simulink model "Project_microgrid_2018a"  (Simulink 9.1)
settings: Solver=VariableStepAuto  StartTime=0.0  StopTime=0.3  RelTol=1e-3
undefined symbols (not defined in the file): D1, D11, Delta, DiscIntNeverNeededParam, find_system, Hydride, Metal, Nickel
libraries: powerlib x104, powerlib_meascontrol x31, sps_avr x14, simulink_extras x4, simulink x3, spsDieselMotorModel x2, electricdrivelib x1, re_lib x1
(part 2 of 5)

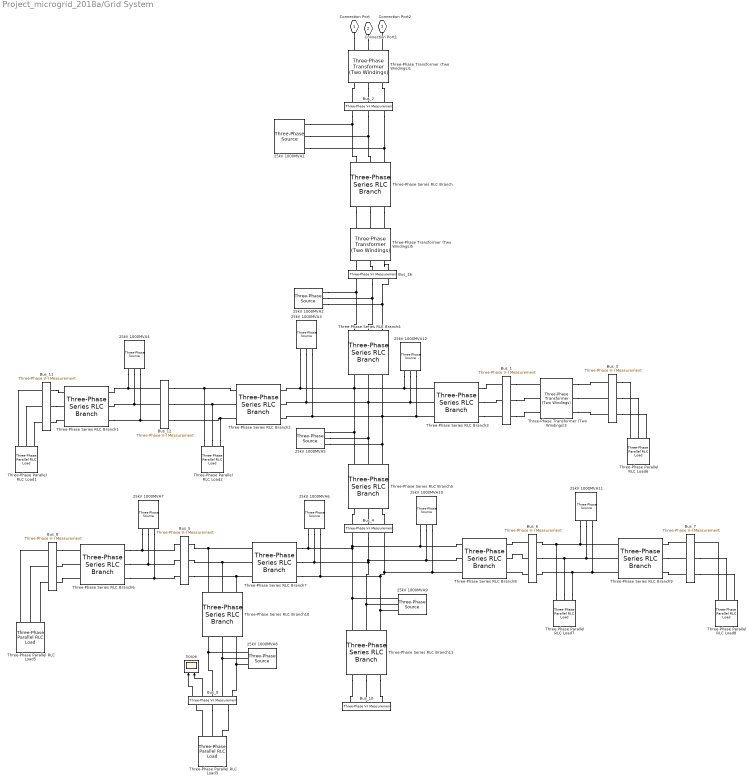
== system Project_microgrid_2018a/Grid System ==
  25kV 1000MVA{1..4,6..12} (11 alike) : powerlib/Electrical Sources/Three-Phase Source  InternalConnection=Yg  VoltagePhases=off  Voltage=10  PhaseAngle=0  Voltage_phases=[25e3 25e3 25e3]/sqrt(3)  PhaseAngles_phases=[0 -120 +120]  Frequency=50  NonIdealSource=on  SpecifyImpedance=on  Resistance=25^2/1000/10  Inductance=25^2/1000/377  ShortCircuitLevel=1000e6  BaseVoltage=25e3  XRratio=10  BusType=swing  Pref=10e3  Qref=0  Prefabc=[10e3, 10e3, 10e3]  Qrefabc=[0, 0, 0]  Qmin=-inf  Qmax=inf
      settings: SourceProductName=Simscape Electrical
  25kV 1000MVA5 : powerlib/Electrical Sources/Three-Phase Source  InternalConnection=Yg  VoltagePhases=off  Voltage=25e3  PhaseAngle=0  Voltage_phases=[25e3 25e3 25e3]/sqrt(3)  PhaseAngles_phases=[0 -120 +120]  Frequency=50  NonIdealSource=on  SpecifyImpedance=on  Resistance=25^2/1000/10  Inductance=25^2/1000/377  ShortCircuitLevel=1000e6  BaseVoltage=25e3  XRratio=10  BusType=swing  Pref=10e3  Qref=0  Prefabc=[10e3, 10e3, 10e3]  Qrefabc=[0, 0, 0]  Qmin=-inf  Qmax=inf
      settings: SourceProductName=Simscape Electrical
  Bus_1 : powerlib/Measurements/Three-Phase V-I Measurement  VoltageMeasurement=phase-to-phase  SetLabelV=on  LabelV=Vabc_5  Vpu=off  VpuLL=off  CurrentMeasurement=yes  SetLabelI=on  LabelI=Iabc_5  Ipu=off  Pbase=100e6  Vbase=120e3  OutputType=Complex  PhasorSimulation=on  PSBequivalent=0
      settings: SourceProductName=Simscape Electrical
  Bus_10 : powerlib/Measurements/Three-Phase V-I Measurement  VoltageMeasurement=phase-to-phase  SetLabelV=on  LabelV=Vabc_13  Vpu=off  VpuLL=off  CurrentMeasurement=yes  SetLabelI=on  LabelI=Iabc_13  Ipu=off  Pbase=100e6  Vbase=120e3  OutputType=Complex  PhasorSimulation=on  PSBequivalent=0
      settings: SourceProductName=Simscape Electrical
  Bus_11 : powerlib/Measurements/Three-Phase V-I Measurement  VoltageMeasurement=phase-to-phase  SetLabelV=on  LabelV=Vabc_3  Vpu=off  VpuLL=off  CurrentMeasurement=yes  SetLabelI=on  LabelI=Iabc_3  Ipu=off  Pbase=100e6  Vbase=120e3  OutputType=Complex  PhasorSimulation=on  PSBequivalent=0
      settings: SourceProductName=Simscape Electrical
  Bus_12 : powerlib/Measurements/Three-Phase V-I Measurement  VoltageMeasurement=phase-to-phase  SetLabelV=on  LabelV=Vabc_4  Vpu=off  VpuLL=off  CurrentMeasurement=yes  SetLabelI=on  LabelI=Iabc_4  Ipu=off  Pbase=100e6  Vbase=120e3  OutputType=Complex  PhasorSimulation=on  PSBequivalent=0
      settings: SourceProductName=Simscape Electrical
  Bus_16 : powerlib/Measurements/Three-Phase V-I Measurement  VoltageMeasurement=phase-to-phase  SetLabelV=on  LabelV=Vabc_1  Vpu=off  VpuLL=off  CurrentMeasurement=yes  SetLabelI=on  LabelI=Iabc_1  Ipu=off  Pbase=100e6  Vbase=120e3  OutputType=Complex  PhasorSimulation=on  PSBequivalent=0
      settings: SourceProductName=Simscape Electrical
  Bus_2 : powerlib/Measurements/Three-Phase V-I Measurement  VoltageMeasurement=phase-to-phase  SetLabelV=on  LabelV=Vabc_2  Vpu=off  VpuLL=off  CurrentMeasurement=yes  SetLabelI=on  LabelI=Iabc_2  Ipu=off  Pbase=100e6  Vbase=120e3  OutputType=Complex  PhasorSimulation=on  PSBequivalent=0
      settings: SourceProductName=Simscape Electrical
  Bus_3 : powerlib/Measurements/Three-Phase V-I Measurement  VoltageMeasurement=phase-to-phase  SetLabelV=on  LabelV=Vabc_6  Vpu=off  VpuLL=off  CurrentMeasurement=yes  SetLabelI=on  LabelI=Iabc_6  Ipu=off  Pbase=100e6  Vbase=120e3  OutputType=Complex  PhasorSimulation=on  PSBequivalent=0
      settings: SourceProductName=Simscape Electrical
  Bus_4 : powerlib/Measurements/Three-Phase V-I Measurement  VoltageMeasurement=phase-to-phase  SetLabelV=on  LabelV=Vabc_7  Vpu=off  VpuLL=off  CurrentMeasurement=yes  SetLabelI=on  LabelI=Iabc_7  Ipu=off  Pbase=100e6  Vbase=120e3  OutputType=Complex  PhasorSimulation=on  PSBequivalent=0
      settings: SourceProductName=Simscape Electrical
  Bus_5 : powerlib/Measurements/Three-Phase V-I Measurement  VoltageMeasurement=phase-to-phase  SetLabelV=on  LabelV=Vabc_8  Vpu=off  VpuLL=off  CurrentMeasurement=yes  SetLabelI=on  LabelI=Iabc_8  Ipu=off  Pbase=100e6  Vbase=120e3  OutputType=Complex  PhasorSimulation=on  PSBequivalent=0
      settings: SourceProductName=Simscape Electrical
  Bus_6 : powerlib/Measurements/Three-Phase V-I Measurement  VoltageMeasurement=phase-to-phase  SetLabelV=on  LabelV=Vabc_10  Vpu=off  VpuLL=off  CurrentMeasurement=yes  SetLabelI=on  LabelI=Iabc_10  Ipu=off  Pbase=100e6  Vbase=120e3  OutputType=Complex  PhasorSimulation=on  PSBequivalent=0
      settings: SourceProductName=Simscape Electrical
  Bus_7 : powerlib/Measurements/Three-Phase V-I Measurement  VoltageMeasurement=phase-to-phase  SetLabelV=on  LabelV=Vabc_11  Vpu=off  VpuLL=off  CurrentMeasurement=yes  SetLabelI=on  LabelI=Iabc_11  Ipu=off  Pbase=100e6  Vbase=120e3  OutputType=Complex  PhasorSimulation=on  PSBequivalent=0
      settings: SourceProductName=Simscape Electrical
  Bus_8 : powerlib/Measurements/Three-Phase V-I Measurement  VoltageMeasurement=phase-to-phase  SetLabelV=on  LabelV=Vabc_9  Vpu=off  VpuLL=off  CurrentMeasurement=yes  SetLabelI=on  LabelI=Iabc_9  Ipu=off  Pbase=100e6  Vbase=120e3  OutputType=Complex  PhasorSimulation=on  PSBequivalent=0
      settings: SourceProductName=Simscape Electrical
  Bus_9 : powerlib/Measurements/Three-Phase V-I Measurement  VoltageMeasurement=phase-to-phase  SetLabelV=off  LabelV=Vabc_12  Vpu=off  VpuLL=off  CurrentMeasurement=yes  SetLabelI=off  LabelI=Iabc_12  Ipu=off  Pbase=100e6  Vbase=120e3  OutputType=Complex  PhasorSimulation=on  PSBequivalent=0
      settings: SourceProductName=Simscape Electrical
  Scope : Scope  NumInputPorts=2
  Three-Phase Parallel RLC Load{1..3,5..8} (7 alike) : powerlib/Elements/Three-Phase Parallel RLC Load  LConnTagsString=A|B|C  Configuration=Y (grounded)  NominalVoltage=415  Vabc=[1e3 1e3 1e3]  Vabcp=[1e3 1e3 1e3]  NominalFrequency=50  UnbalancedPower=off  ActivePower=10e3  InductivePower=0  CapacitivePower=0  Pabc=[10e3 9e3 11e3]  QLabc=[100 90 110]  QCabc=[100 90 110]  Pabcp=[10e3 9e3 11e3]  QLabcp=[100 90 110]  QCabcp=[100 90 110]  Measurements=None  LoadType=constant Z
      settings: SourceProductName=Simscape Electrical
  Three-Phase Series RLC Branch{,1..11} (12 alike) : powerlib/Elements/Three-Phase Series RLC Branch  LConnTagsString=A|B|C  RConnTagsString=A|B|C  BranchType=RL  Resistance=10  Inductance=1e-3  Capacitance=1e-6  Measurements=None
      settings: SourceProductName=Simscape Electrical
  Three-Phase Transformer (Two Windings)1 : powerlib/Elements/Three-Phase Transformer (Two Windings)  Winding1Connection=Delta (D1)  Winding2Connection=Yg  CoreType=Three single-phase transformers  SetSaturation=off  Hysteresis=off  DataFile='hysteresis'  SetInitialFlux=off  Measurements=None  UNITS=pu  NominalPower=[ 1 , 50 ]  Winding1=[ 1.06 , 0.002 , 0.08 ]  Winding2=[100 , 0.002 , 0.08 ]  Rm=500  Lm=500  L0=0.5  Saturation=[ 0,0 ; 0.0024,1.2 ; 1.0,1.52 ]  InitialFluxes=[ 0.8 , -0.8 , 0.7 ]  BreakLoop=off  DiscreteSolver=Trapezoidal iterative  DataType=off  TransfoNumber=1
      settings: SourceProductName=Simscape Electrical
  Three-Phase Transformer (Two Windings)3 : powerlib/Elements/Three-Phase Transformer (Two Windings)  Winding1Connection=Delta (D1)  Winding2Connection=Yg  CoreType=Three single-phase transformers  SetSaturation=off  Hysteresis=off  DataFile='hysteresis'  SetInitialFlux=off  Measurements=None  UNITS=pu  NominalPower=[ 1 , 50 ]  Winding1=[ 1.06 , 0.002 , 0.08 ]  Winding2=[ 1.06 , 0.002 , 0.08 ]  Rm=500  Lm=500  L0=0.5  Saturation=[ 0,0 ; 0.0024,1.2 ; 1.0,1.52 ]  InitialFluxes=[ 0.8 , -0.8 , 0.7 ]  BreakLoop=off  DiscreteSolver=Trapezoidal iterative  DataType=off  TransfoNumber=1
      settings: SourceProductName=Simscape Electrical
  Three-Phase Transformer (Two Windings)5 : powerlib/Elements/Three-Phase Transformer (Two Windings)  Winding1Connection=Delta (D1)  Winding2Connection=Yg  CoreType=Three single-phase transformers  SetSaturation=off  Hysteresis=off  DataFile='hysteresis'  SetInitialFlux=off  Measurements=None  UNITS=pu  NominalPower=[ 1 , 50 ]  Winding1=[ 1.06 , 0.002 , 0.08 ]  Winding2=[1000 , 0.002 , 0.08 ]  Rm=500  Lm=500  L0=0.5  Saturation=[ 0,0 ; 0.0024,1.2 ; 1.0,1.52 ]  InitialFluxes=[ 0.8 , -0.8 , 0.7 ]  BreakLoop=off  DiscreteSolver=Trapezoidal iterative  DataType=off  TransfoNumber=1
      settings: SourceProductName=Simscape Electrical
  Connection Port : PMIOPort  Tag=PMCPort  Side=Left
  Connection Port1 : PMIOPort  Tag=PMCPort  Port=2  Side=Left
  Connection Port2 : PMIOPort  Tag=PMCPort  Port=3  Side=Left
  wires:
  Bus_9/1 -> Scope/1
  Bus_9/2 -> Scope/2
  connections:
  Three-Phase Parallel RLC Load2/LConn3 -- Bus_12/RConn3 -- Three-Phase Series RLC Branch2/LConn3
  Three-Phase Parallel RLC Load2/LConn2 -- Three-Phase Series RLC Branch2/LConn2 -- Bus_12/RConn2
  Three-Phase Parallel RLC Load2/LConn1 -- Bus_12/RConn1 -- Three-Phase Series RLC Branch2/LConn1
  Three-Phase Series RLC Branch10/RConn2 -- Bus_5/RConn2 -- Three-Phase Series RLC Branch7/LConn2
  Three-Phase Series RLC Branch10/RConn3 -- Bus_5/RConn3 -- Three-Phase Series RLC Branch7/LConn3
  Three-Phase Series RLC Branch10/RConn1 -- Bus_5/RConn1 -- Three-Phase Series RLC Branch7/LConn1
  25kV 1000MVA12/RConn1 -- Three-Phase Series RLC Branch4/RConn1 -- Three-Phase Series RLC Branch2/RConn1 -- 25kV 1000MVA3/RConn1 -- Three-Phase Series RLC Branch5/LConn1 -- 25kV 1000MVA5/RConn1 -- Three-Phase Series RLC Branch3/LConn1
  25kV 1000MVA12/RConn2 -- Three-Phase Series RLC Branch2/RConn2 -- 25kV 1000MVA3/RConn2 -- Three-Phase Series RLC Branch4/RConn2 -- Three-Phase Series RLC Branch5/LConn2 -- 25kV 1000MVA5/RConn2 -- Three-Phase Series RLC Branch3/LConn2
  25kV 1000MVA12/RConn3 -- Three-Phase Series RLC Branch4/RConn3 -- Three-Phase Series RLC Branch2/RConn3 -- 25kV 1000MVA3/RConn3 -- Three-Phase Series RLC Branch5/LConn3 -- 25kV 1000MVA5/RConn3 -- Three-Phase Series RLC Branch3/LConn3
  25kV 1000MVA10/RConn1 -- Three-Phase Series RLC Branch7/RConn1 -- 25kV 1000MVA6/RConn1 -- Three-Phase Series RLC Branch11/LConn1 -- 25kV 1000MVA9/RConn1 -- Bus_4/LConn1 -- Three-Phase Series RLC Branch8/LConn1
  25kV 1000MVA10/RConn2 -- Three-Phase Series RLC Branch7/RConn2 -- 25kV 1000MVA6/RConn2 -- Three-Phase Series RLC Branch11/LConn2 -- 25kV 1000MVA9/RConn2 -- Bus_4/LConn2 -- Three-Phase Series RLC Branch8/LConn2
  25kV 1000MVA10/RConn3 -- Bus_4/LConn3 -- Three-Phase Series RLC Branch7/RConn3 -- 25kV 1000MVA6/RConn3 -- Three-Phase Series RLC Branch11/LConn3 -- 25kV 1000MVA9/RConn3 -- Three-Phase Series RLC Branch8/LConn3
  25kV 1000MVA4/RConn3 -- Three-Phase Series RLC Branch1/RConn3 -- Bus_12/LConn3
  25kV 1000MVA1/RConn3 -- Bus_2/LConn3 -- Three-Phase Series RLC Branch/LConn3
  25kV 1000MVA8/RConn3 -- Bus_9/RConn3 -- Three-Phase Series RLC Branch10/LConn3
  Three-Phase Parallel RLC Load7/LConn1 -- Bus_6/RConn1 -- Three-Phase Series RLC Branch9/LConn1 -- 25kV 1000MVA11/RConn1
  25kV 1000MVA4/RConn1 -- Three-Phase Series RLC Branch1/RConn1 -- Bus_12/LConn1
  25kV 1000MVA2/RConn2 -- Bus_16/LConn2 -- Three-Phase Series RLC Branch4/LConn2
  25kV 1000MVA2/RConn3 -- Bus_16/LConn3 -- Three-Phase Series RLC Branch4/LConn3
  25kV 1000MVA8/RConn1 -- Bus_9/RConn1 -- Three-Phase Series RLC Branch10/LConn1
  25kV 1000MVA2/RConn1 -- Bus_16/LConn1 -- Three-Phase Series RLC Branch4/LConn1
  25kV 1000MVA4/RConn2 -- Three-Phase Series RLC Branch1/RConn2 -- Bus_12/LConn2
  25kV 1000MVA7/RConn1 -- Three-Phase Series RLC Branch6/RConn1 -- Bus_5/LConn1
  Three-Phase Parallel RLC Load7/LConn2 -- Bus_6/RConn2 -- Three-Phase Series RLC Branch9/LConn2 -- 25kV 1000MVA11/RConn2
  25kV 1000MVA8/RConn2 -- Bus_9/RConn2 -- Three-Phase Series RLC Branch10/LConn2
  25kV 1000MVA1/RConn2 -- Bus_2/LConn2 -- Three-Phase Series RLC Branch/LConn2
  25kV 1000MVA1/RConn1 -- Bus_2/LConn1 -- Three-Phase Series RLC Branch/LConn1
  25kV 1000MVA7/RConn2 -- Three-Phase Series RLC Branch6/RConn2 -- Bus_5/LConn2
  25kV 1000MVA7/RConn3 -- Three-Phase Series RLC Branch6/RConn3 -- Bus_5/LConn3
  Three-Phase Parallel RLC Load7/LConn3 -- Bus_6/RConn3 -- Three-Phase Series RLC Branch9/LConn3 -- 25kV 1000MVA11/RConn3
  Three-Phase Series RLC Branch/RConn1 -- Three-Phase Transformer (Two Windings)5/LConn1
  Bus_7/RConn2 -- Three-Phase Parallel RLC Load8/LConn2
  Three-Phase Parallel RLC Load1/LConn2 -- Bus_11/LConn2
  Three-Phase Series RLC Branch5/RConn3 -- Bus_4/RConn3
  Three-Phase Transformer (Two Windings)3/LConn3 -- Bus_3/LConn3
  Bus_6/LConn2 -- Three-Phase Series RLC Branch8/RConn2
  Bus_1/RConn2 -- Three-Phase Transformer (Two Windings)3/RConn2
  Bus_11/RConn3 -- Three-Phase Series RLC Branch1/LConn3
  Bus_6/LConn3 -- Three-Phase Series RLC Branch8/RConn3
  Bus_8/RConn2 -- Three-Phase Series RLC Branch6/LConn2
  Three-Phase Parallel RLC Load5/LConn2 -- Bus_8/LConn2
  Three-Phase Series RLC Branch/RConn3 -- Three-Phase Transformer (Two Windings)5/LConn3
  Bus_7/RConn3 -- Three-Phase Parallel RLC Load8/LConn3
  Bus_3/RConn1 -- Three-Phase Parallel RLC Load6/LConn1
  Three-Phase Parallel RLC Load8/LConn1 -- Bus_7/RConn1
  Three-Phase Parallel RLC Load5/LConn1 -- Bus_8/LConn1
  Three-Phase Series RLC Branch11/RConn1 -- Bus_10/RConn1
  Three-Phase Transformer (Two Windings)1/RConn3 -- Bus_2/RConn3
  Three-Phase Series RLC Branch9/RConn2 -- Bus_7/LConn2
  Bus_11/RConn2 -- Three-Phase Series RLC Branch1/LConn2
  Three-Phase Series RLC Branch3/RConn3 -- Bus_1/LConn3
  Bus_9/LConn2 -- Three-Phase Parallel RLC Load3/LConn2
  Three-Phase Transformer (Two Windings)3/LConn1 -- Bus_3/LConn1
  Three-Phase Series RLC Branch3/RConn1 -- Bus_1/LConn1
  Three-Phase Parallel RLC Load5/LConn3 -- Bus_8/LConn3
  Three-Phase Parallel RLC Load1/LConn3 -- Bus_11/LConn3
  Three-Phase Transformer (Two Windings)5/RConn2 -- Bus_16/RConn2
  Three-Phase Series RLC Branch3/RConn2 -- Bus_1/LConn2
  Three-Phase Series RLC Branch9/RConn3 -- Bus_7/LConn3
  Bus_9/LConn3 -- Three-Phase Parallel RLC Load3/LConn3
  Bus_6/LConn1 -- Three-Phase Series RLC Branch8/RConn1
  Bus_1/RConn3 -- Three-Phase Transformer (Two Windings)3/RConn3
  Bus_4/RConn2 -- Three-Phase Series RLC Branch5/RConn2
  Bus_3/RConn3 -- Three-Phase Parallel RLC Load6/LConn3
  Bus_8/RConn3 -- Three-Phase Series RLC Branch6/LConn3
  Three-Phase Series RLC Branch11/RConn2 -- Bus_10/RConn2
  Bus_1/RConn1 -- Three-Phase Transformer (Two Windings)3/RConn1
  Three-Phase Series RLC Branch11/RConn3 -- Bus_10/RConn3
  Three-Phase Transformer (Two Windings)3/LConn2 -- Bus_3/LConn2
  Three-Phase Transformer (Two Windings)1/RConn2 -- Bus_2/RConn2
  Bus_3/RConn2 -- Three-Phase Parallel RLC Load6/LConn2
  Three-Phase Transformer (Two Windings)5/RConn1 -- Bus_16/RConn1
  Three-Phase Series RLC Branch9/RConn1 -- Bus_7/LConn1
  Three-Phase Parallel RLC Load3/LConn1 -- Bus_9/LConn1
  Bus_11/RConn1 -- Three-Phase Series RLC Branch1/LConn1
  Three-Phase Parallel RLC Load1/LConn1 -- Bus_11/LConn1
  Bus_4/RConn1 -- Three-Phase Series RLC Branch5/RConn1
  Three-Phase Transformer (Two Windings)1/RConn1 -- Bus_2/RConn1
  Three-Phase Series RLC Branch/RConn2 -- Three-Phase Transformer (Two Windings)5/LConn2
  Three-Phase Transformer (Two Windings)5/RConn3 -- Bus_16/RConn3
  Connection Port1/RConn1 -- Three-Phase Transformer (Two Windings)1/LConn2
  Bus_8/RConn1 -- Three-Phase Series RLC Branch6/LConn1
  Connection Port/RConn1 -- Three-Phase Transformer (Two Windings)1/LConn1
  Connection Port2/RConn1 -- Three-Phase Transformer (Two Windings)1/LConn3

== system Project_microgrid_2018a/Inveter ==
  3-Level Bridge : powerlib/Power Electronics/Three-Level Bridge  Arms=3  SnubberResistance=1e6  SbubberCapacitance=inf  Device=IGBT / Diodes  Ron=0.2e-3  ForwardVoltages="[  0  0 ]"  Measurements=None
      settings: SourceProductName=Simscape Electrical  SourceProductBaseCode=PS
  VSC Contoler : Subsystem
  +Vin : PMIOPort  Side=Right
  A : PMIOPort  Port=2  Side=Left
  N : PMIOPort  Port=3  Side=Right
  B : PMIOPort  Port=4  Side=Left
  -Vin : PMIOPort  Port=5  Side=Right
  C : PMIOPort  Port=6  Side=Left
  wires:
  VSC Contoler/1(Inveter Pulse) -> 3-Level Bridge/1
  connections:
  3-Level Bridge/RConn1 -- +Vin/RConn1
  3-Level Bridge/RConn3 -- -Vin/RConn1
  3-Level Bridge/LConn1 -- A/RConn1
  3-Level Bridge/RConn2 -- N/RConn1
  3-Level Bridge/LConn3 -- C/RConn1
  3-Level Bridge/LConn2 -- B/RConn1

== system Project_microgrid_2018a/MPPT Controler  ==
  Delay : Delay  DelayLength=1
  Delay1 : Delay  DelayLength=1
  Delay2 : Delay  DelayLength=1
  MATLAB Function : MATLAB Function  TreatAsAtomicUnit=on
  Relational Operator : RelationalOperator  Operator=<=  OutDataTypeStr=boolean  RndMeth=Simplest
  Repeating Sequence : simulink/Sources/Repeating Sequence  rep_seq_t=[0 0.5 1]/1000  rep_seq_y=[0 1 0]
  Boost Conveter Pulse : Outport
  wires:
  [I_PV] -> Delay1/1, MATLAB Function/3(I)
  MATLAB Function/1(D) -> Relational Operator/2, Delay2/1
  [V_PV] -> Delay/1, MATLAB Function/1(V)
  Delay/1 -> MATLAB Function/2(v)
  Delay1/1 -> MATLAB Function/4(i)
  Delay2/1 -> MATLAB Function/5(d)
  Relational Operator/1 -> Boost Conveter Pulse/1
  Repeating Sequence/1 -> Relational Operator/1

== system Project_microgrid_2018a/PV System  ==
  Bus Selector : BusSelector  OutputSignals=V_PV,I_PV,I_diode,Irradiance (W/m2),Temperature (deg C)
  Delay : Delay  DelayLength=1
  Step : Step  After=1000  SampleTime=0
  Temp : Constant  Value=25  SampleTime=1e-6
  Transparent PV Array : re_lib/Solar/PV Array  Npar=6  Nser=5  PlotType=array @ 1000 W/m2 & specified temperatures  S_vec="[ 1000  250 ]"  Temp_C_vec="[0 25 50  ]"  ModuleName=User-defined  PlotWhenSelected=off  Pm=244.9746  Ncell=96  Voc=40.53  Isc=7.66  Vm=33.93  Im=7.22  beta_Voc_pc=-0.35  alpha_Isc_pc=0.04  beta_Voc=-0.14185  alpha_Isc=0.003064  IL=7.7674  I0=1.7813e-10  nI=0.67155  Rsh=182.6307  Rs=0.21635  BAL=on  Tc=Tc  Tfilter=5e-5
      settings: SourceProductName=Simscape Electrical
  V+ : PMIOPort  Side=Right
  V- : PMIOPort  Port=2  Side=Right
  tag scope: I_PV=global, Idiode_PV=global, Ir=global, Temp=global, V_PV=global
  wires:
  Bus Selector/3 -> [Idiode_PV]  "<I_diode>"
  Bus Selector/5 -> [Temp]  "<Temperature (deg C)>"
  Bus Selector/1 -> [V_PV]  "<V_PV>"
  Bus Selector/2 -> [I_PV]  "<I_PV>"
  Bus Selector/4 -> [Ir]  "<Irradiance (W/m2)>"
  Transparent PV Array/1 -> Bus Selector/1
  Delay/1 -> Transparent PV Array/1
  Step/1 -> Delay/1
  Temp/1 -> Transparent PV Array/2
  connections:
  V+/RConn1 -- Transparent PV Array/RConn1
  V-/RConn1 -- Transparent PV Array/RConn2

== system Project_microgrid_2018a/Relay G ==
  AC Time Overcurrent Relay2 : Subsystem  mask(AC Time Overcurrent Relay Block){tcpopup=Definite Minimum Time, k=0, alpha=0.02, B=0, PS=100%, TMS=0.1, TDS=5, CTpri=300, CTsec=5, Freq=60, RMSInit=0}
      mask prompts: tcpopup "Trip Characteristic"; PS "Plug Setting (PS) / Low-set (I >)"; TMS "Time Multiplier Setting (TMS)"; TDS "Time Delay Setting (TDS) in sec"; CTpri "Current Transformer Primary (A)"; CTsec "Current Transformer Secondary (A)"; Freq "Fundamental frequency (Hz):"; RMSInit "Initial RMS value:"
      mask help:
      | AC Time Overcurrent Relay Block developed by Dr Rodney Tan
      | Version 1.0 (Jun 2016)
      |
      | AC Time Overcurrent Relay (ANSI/IEEE C37.2 device number 51) that operates when the current exceeds a predetermined value.
      |
      | This relay operates with either a Definite Minimum Time (DMT) or Inverse Definite Minimum Time (IDMT) characteristic.
      |
      | This relay support both IEC 60255 Standard and IEEE Standard C37.112-1996 IDMT trip characteristic.
      mask Help:
      | <b><u>Block Setting</u></b>
      | <b>Trip Characteristic</b>
      | Relay operation mode selection of Definite Minimum Time (DMT), IEC 60255 Standard or IEEE Standard C37.112-1996 Inverse Definite Minimum Time (IDMT).
      | 
      | <b>Plug-Setting(PS) / Low-set (I >)</b>
      | Specify relay pick-up current based on current transformer rating ranging from 25% to 200% with 25% step interval.
      | 
      | <b>Time Multiplier Setting (TMS)</b>
      | Specify time delay multiplier ranging from 0.05 to 1.0 for IDMT relay operation. This setting will be disabled DMT relay operation mode.
      | 
      | <b>Plot Curve Button</b>
      | Plot current Inverse Definite Minimum Time trip curve.
      | 
      | <b>Time Delay Setting (TDS)</b>
      | Specify time delay ranging from 0.05sec to 99sec for Definite Minimum Time relay operation. This setting will be disabled in IDMT relay operation mode.
      | 
      | <b>Current Transformer Primary (A)</b>
      | Specify current transformer primary in Ampere.
      | 
      | <b>Current Transformer Secondary (A)</b>
      | Specify current transformer secondary in Ampere.
      | 
      | <b>Fundamental Frequency (Hz)</b>
      | Specify the RMS current measurement fundamental frequency, in hertz, of the input signal.
      | 
      | <b>Initial RMS Value</b>
      | Specify the RMS current measurement initial RMS value of the output signal.
      | 
      | <b><u>Block Input Output</u></b>
      | <b>I</b>
      | Current input to the AC time overcurrent relay
      | 
      | <b>trip</b>
      | Trip control signal output (1-0), commonly connected to circuit breaker
      | 
      | <b>OT</b>
      | Relay operating time output
      mask TypeOptions tcpopup: Definite Minimum Time | IEC Standard Inverse | IEC Very Inverse | IEC Long Time Inverse | IEC Extremely Inverse | IEC Ultra Inverse | IEEE Moderately Inverse | IEEE Very Inverse | IEEE Extremely Inverse
      mask Callback tcpopup:
      | switch(get_param(gcb,'tcpopup'))
      |     case 'IEC Standard Inverse'
      |         set_param(gcb,'k','0.14');
      |         set_param(gcb,'alpha','0.02');
      |         set_param(gcb,'B','0');
      |         set_param(gcb,'MaskEnables',{'on','off','off','off',...
      |                   'on','on','off','on','on','on','on'});
      |     case 'IEC Very Inverse'
      |         set_param(gcb,'k','13.5');
      |         set_param(gcb,'alpha','1');
      |         set_param(gcb,'B','0');
      |         set_param(gcb,'MaskEnables',{'on','off','off','off',...
      |                   'on','on','off','on','on','on','on'});
      |     case 'IEC Long Time Inverse'
      |         set_param(gcb,'k','120');
      |         set_param(gcb,'alpha','1');
      |         set_param(gcb,'B','0');
      |         set_param(gcb,'MaskEnables',{'on','off','off','off',...
      |                   'on','on','off','on','on','on','on'});
      |     case 'IEC Extremely Inverse'
      |         set_param(gcb,'k','80');
      |         set_param(gcb,'alpha','2');
      |         set_param(gcb,'B','0');
      |         set_param(gcb,'MaskEnables',{'on','off','off','off',...
      |                   'on','on','off','on','on','on','on'});
      |     case 'IEC Ultra Inverse'
      |         set_param(gcb,'k','315.2');
      |         set_param(gcb,'alpha','2.5');
      |         set_param(gcb,'B','0');
      |         set_param(gcb,'MaskEnables',{'on','off','off','off',...
      |                   'on','on','off','on','on','on','on'});
      |     case 'IEEE Moderately Inverse'
      |         set_param(gcb,'k','0.0515');
      |         set_param(gcb,'alpha','0.02');
      |         set_param(gcb,'B','0.114');
      |         set_param(gcb,'MaskEnables',{'on','off','off','off',...
      |                   'on','on','off','on','on','on','on'});
      |     case 'IEEE Very Inverse'
      |         set_param(gcb,'k','19.61');
      |         set_param(gcb,'alpha','2');
      |         set_param(gcb,'B','0.491');
      |         set_param(gcb,'MaskEnables',{'on','off','off','off',...
      |                   'on','on','off','on','on','on','on'});
      |     case 'IEEE Extremely Inverse'
      |         set_param(gcb,'k','28.2');
      |         set_param(gcb,'alpha','2');
      |         set_param(gcb,'B','0.1217');
      |         set_param(gcb,'MaskEnables',{'on','off','off','off',...
      |                   'on','on','off','on','on','on','on'});
      |     otherwise
      |         set_param(gcb,'k','0');
      |         set_param(gcb,'MaskEnables',{'on','off','off','off',...
      |                   'on','off','on','on','on','on','on'});
      | end
      mask TypeOptions PS: 25% | 50% | 75% | 100% | 125% | 150% | 175% | 200%
      mask TypeOptions TMS: 0.05 | 0.1 | 0.15 | 0.2 | 0.25 | 0.3 | 0.35 | 0.4 | 0.45 | 0.5 | 0.55 | 0.6 | 0.65 | 0.7 | 0.75 | 0.8 | 0.85 | 0.9 | 0.95 | 1.0
      mask Callback TDS:
      | TDS = str2double(get_param(gcb,'TDS'));
      | if (TDS > 99)||(TDS < 0.05)||isnan(TDS)
      |     msgbox('TDS must be in the range of 0.05-99 sec',...
      |     'Invalid Value !','error');
      |     set_param(gcb,'TDS','0.1');
      | end
      mask TypeOptions Freq: Irms/Freq
      mask TypeOptions RMSInit: Irms/RMSInit
      mask DialogControl plotbutton Prompt: Plot Curve
      mask DialogControl plotbutton Callback:
      | % Plotting IDMT Curve
      | TMS = str2num(get_param(gcb,'TMS'));
      | k = str2num(get_param(gcb,'k'));
      | alpha = str2num(get_param(gcb,'alpha'));
      | B = str2num(get_param(gcb,'B'));
      | I = 1:20;
      | td = ((k./((I.^alpha)-1))+B)*TMS;
      | loglog(td);
      | set(gcf, 'Position', [200 150 300 500]);
      | switch(get_param(gcb,'tcpopup'))
      |     case 'IEC Standard Inverse'
      |         title('IEC Standard Inverse');
      |         set(gca, 'YTick', (1:10));
      |         ylim([0.1 10]);
      |     case 'IEC Very Inverse'
      |         title('IEC Very Inverse');
      |         set(gca, 'YTick', (1:2:15));
      |         ylim([0.01 15]);
      |     case 'IEC Long Time Inverse'
      |         title('IEC Long Time Inverse');
      |         set(gca, 'YTick', (0:20:120));
      |         ylim([0.1 120]);
      |     case 'IEC Extremely Inverse'
      |         title('IEC Extremely Inverse');
      |         set(gca, 'YTick', (0:5:30));
      |         ylim([0.01 30]);
      |     case 'IEC Ultra Inverse'
      |         title('IEC Ultra Inverse');
      |         set(gca, 'YTick', (0:20:100));
      |         ylim([0.01 100]);
      |     case 'IEEE Moderately Inverse'
      |         title('IEEE Moderately Inverse');
      |         set(gca, 'YTick', (1:5));
      |         ylim([0.01 5]);
      |     case 'IEEE Very Inverse'
      |         title('IEEE Very Inverse');
      |         set(gca, 'YTick', (1:10));
      |         ylim([0.01 10]);
      |     case 'IEEE Extremely Inverse'
      |         title('IEEE Extremely Inverse');
      |         set(gca, 'YTick', (1:10));
      |         ylim([0.01 10]);
      | end
      | 
      | set(gca, 'XTick', [1:10 20]);
      | xlim([1 30]);
      | xlabel('Current (Multiples of Plug Setting)');
      | ylabel('Operating Time (sec)');
      | grid on;
      mask DialogControl RMS Prompt: RMS Current Measurement
      mask Display:
      | disp('(51)');
      | port_label('input', 1, 'I');
      | port_label('output', 1, 'trip');
      | port_label('output', 2, 'OT');
  Display : Display
  Output1 : Subsystem
  Three-Phase V-I Measurement : powerlib/Measurements/Three-Phase V-I Measurement  VoltageMeasurement=no  SetLabelV=off  LabelV=Vabc  Vpu=off  VpuLL=off  CurrentMeasurement=yes  SetLabelI=off  LabelI=Iabc  Ipu=off  Pbase=100e6  Vbase=500e3  OutputType=Complex  PhasorSimulation=off  PSBequivalent=0
      settings: SourceProductName=Simscape Electrical
  Three-Phase Breaker : powerlib/Elements/Three-Phase Breaker  InitialState=closed  SwitchA=on  SwitchB=on  SwitchC=on  SwitchTimes="[1/60  5/60]"  External=on  BreakerResistance=0.001  SnubberResistance=1e6  SnubberCapacitance=inf  Measurements=None
      settings: SourceProductName=Simscape Electrical
  A : PMIOPort  Side=Left
  a : PMIOPort  Port=2  Side=Right
  B : PMIOPort  Port=3  Side=Left
  b : PMIOPort  Port=4  Side=Right
  C : PMIOPort  Port=5  Side=Left
  c : PMIOPort  Port=6  Side=Right
  tag scope: G_B=global
  wires:
  Three-Phase V-I Measurement/1 -> Output1/1(Signal), AC Time Overcurrent Relay2/1(I)  "Iabc"
  AC Time Overcurrent Relay2/2(OT) -> Display/1
  AC Time Overcurrent Relay2/1(C.B) -> [G_B], Three-Phase Breaker/1  "Relay C"
  connections:
  Three-Phase Breaker/RConn2 -- Three-Phase V-I Measurement/LConn2
  Three-Phase V-I Measurement/RConn2 -- b/RConn1
  Three-Phase V-I Measurement/LConn1 -- Three-Phase Breaker/RConn1
  Three-Phase Breaker/LConn2 -- B/RConn1
  Three-Phase V-I Measurement/RConn1 -- a/RConn1
  Three-Phase Breaker/RConn3 -- Three-Phase V-I Measurement/LConn3
  Three-Phase Breaker/LConn3 -- C/RConn1
  Three-Phase V-I Measurement/RConn3 -- c/RConn1
  Three-Phase Breaker/LConn1 -- A/RConn1

== system Project_microgrid_2018a/Relay PV ==
  AC Time Overcurrent Relay2 : Subsystem  mask(AC Time Overcurrent Relay Block){tcpopup=Definite Minimum Time, k=0, alpha=0.02, B=0, PS=100%, TMS=0.1, TDS=5, CTpri=300, CTsec=5, Freq=60, RMSInit=0}
      mask prompts: tcpopup "Trip Characteristic"; PS "Plug Setting (PS) / Low-set (I >)"; TMS "Time Multiplier Setting (TMS)"; TDS "Time Delay Setting (TDS) in sec"; CTpri "Current Transformer Primary (A)"; CTsec "Current Transformer Secondary (A)"; Freq "Fundamental frequency (Hz):"; RMSInit "Initial RMS value:"
      mask help:
      | AC Time Overcurrent Relay Block developed by Dr Rodney Tan
      | Version 1.0 (Jun 2016)
      |
      | AC Time Overcurrent Relay (ANSI/IEEE C37.2 device number 51) that operates when the current exceeds a predetermined value.
      |
      | This relay operates with either a Definite Minimum Time (DMT) or Inverse Definite Minimum Time (IDMT) characteristic.
      |
      | This relay support both IEC 60255 Standard and IEEE Standard C37.112-1996 IDMT trip characteristic.
      mask Help:
      | <b><u>Block Setting</u></b>
      | <b>Trip Characteristic</b>
      | Relay operation mode selection of Definite Minimum Time (DMT), IEC 60255 Standard or IEEE Standard C37.112-1996 Inverse Definite Minimum Time (IDMT).
      | 
      | <b>Plug-Setting(PS) / Low-set (I >)</b>
      | Specify relay pick-up current based on current transformer rating ranging from 25% to 200% with 25% step interval.
      | 
      | <b>Time Multiplier Setting (TMS)</b>
      | Specify time delay multiplier ranging from 0.05 to 1.0 for IDMT relay operation. This setting will be disabled DMT relay operation mode.
      | 
      | <b>Plot Curve Button</b>
      | Plot current Inverse Definite Minimum Time trip curve.
      | 
      | <b>Time Delay Setting (TDS)</b>
      | Specify time delay ranging from 0.05sec to 99sec for Definite Minimum Time relay operation. This setting will be disabled in IDMT relay operation mode.
      | 
      | <b>Current Transformer Primary (A)</b>
      | Specify current transformer primary in Ampere.
      | 
      | <b>Current Transformer Secondary (A)</b>
      | Specify current transformer secondary in Ampere.
      | 
      | <b>Fundamental Frequency (Hz)</b>
      | Specify the RMS current measurement fundamental frequency, in hertz, of the input signal.
      | 
      | <b>Initial RMS Value</b>
      | Specify the RMS current measurement initial RMS value of the output signal.
      | 
      | <b><u>Block Input Output</u></b>
      | <b>I</b>
      | Current input to the AC time overcurrent relay
      | 
      | <b>trip</b>
      | Trip control signal output (1-0), commonly connected to circuit breaker
      | 
      | <b>OT</b>
      | Relay operating time output
      mask TypeOptions tcpopup: Definite Minimum Time | IEC Standard Inverse | IEC Very Inverse | IEC Long Time Inverse | IEC Extremely Inverse | IEC Ultra Inverse | IEEE Moderately Inverse | IEEE Very Inverse | IEEE Extremely Inverse
      mask Callback tcpopup:
      | switch(get_param(gcb,'tcpopup'))
      |     case 'IEC Standard Inverse'
      |         set_param(gcb,'k','0.14');
      |         set_param(gcb,'alpha','0.02');
      |         set_param(gcb,'B','0');
      |         set_param(gcb,'MaskEnables',{'on','off','off','off',...
      |                   'on','on','off','on','on','on','on'});
      |     case 'IEC Very Inverse'
      |         set_param(gcb,'k','13.5');
      |         set_param(gcb,'alpha','1');
      |         set_param(gcb,'B','0');
      |         set_param(gcb,'MaskEnables',{'on','off','off','off',...
      |                   'on','on','off','on','on','on','on'});
      |     case 'IEC Long Time Inverse'
      |         set_param(gcb,'k','120');
      |         set_param(gcb,'alpha','1');
      |         set_param(gcb,'B','0');
      |         set_param(gcb,'MaskEnables',{'on','off','off','off',...
      |                   'on','on','off','on','on','on','on'});
      |     case 'IEC Extremely Inverse'
      |         set_param(gcb,'k','80');
      |         set_param(gcb,'alpha','2');
      |         set_param(gcb,'B','0');
      |         set_param(gcb,'MaskEnables',{'on','off','off','off',...
      |                   'on','on','off','on','on','on','on'});
      |     case 'IEC Ultra Inverse'
      |         set_param(gcb,'k','315.2');
      |         set_param(gcb,'alpha','2.5');
      |         set_param(gcb,'B','0');
      |         set_param(gcb,'MaskEnables',{'on','off','off','off',...
      |                   'on','on','off','on','on','on','on'});
      |     case 'IEEE Moderately Inverse'
      |         set_param(gcb,'k','0.0515');
      |         set_param(gcb,'alpha','0.02');
      |         set_param(gcb,'B','0.114');
      |         set_param(gcb,'MaskEnables',{'on','off','off','off',...
      |                   'on','on','off','on','on','on','on'});
      |     case 'IEEE Very Inverse'
      |         set_param(gcb,'k','19.61');
      |         set_param(gcb,'alpha','2');
      |         set_param(gcb,'B','0.491');
      |         set_param(gcb,'MaskEnables',{'on','off','off','off',...
      |                   'on','on','off','on','on','on','on'});
      |     case 'IEEE Extremely Inverse'
      |         set_param(gcb,'k','28.2');
      |         set_param(gcb,'alpha','2');
      |         set_param(gcb,'B','0.1217');
      |         set_param(gcb,'MaskEnables',{'on','off','off','off',...
      |                   'on','on','off','on','on','on','on'});
      |     otherwise
      |         set_param(gcb,'k','0');
      |         set_param(gcb,'MaskEnables',{'on','off','off','off',...
      |                   'on','off','on','on','on','on','on'});
      | end
      mask TypeOptions PS: 25% | 50% | 75% | 100% | 125% | 150% | 175% | 200%
      mask TypeOptions TMS: 0.05 | 0.1 | 0.15 | 0.2 | 0.25 | 0.3 | 0.35 | 0.4 | 0.45 | 0.5 | 0.55 | 0.6 | 0.65 | 0.7 | 0.75 | 0.8 | 0.85 | 0.9 | 0.95 | 1.0
      mask Callback TDS:
      | TDS = str2double(get_param(gcb,'TDS'));
      | if (TDS > 99)||(TDS < 0.05)||isnan(TDS)
      |     msgbox('TDS must be in the range of 0.05-99 sec',...
      |     'Invalid Value !','error');
      |     set_param(gcb,'TDS','0.1');
      | end
      mask TypeOptions Freq: Irms/Freq
      mask TypeOptions RMSInit: Irms/RMSInit
      mask DialogControl plotbutton Prompt: Plot Curve
      mask DialogControl plotbutton Callback:
      | % Plotting IDMT Curve
      | TMS = str2num(get_param(gcb,'TMS'));
      | k = str2num(get_param(gcb,'k'));
      | alpha = str2num(get_param(gcb,'alpha'));
      | B = str2num(get_param(gcb,'B'));
      | I = 1:20;
      | td = ((k./((I.^alpha)-1))+B)*TMS;
      | loglog(td);
      | set(gcf, 'Position', [200 150 300 500]);
      | switch(get_param(gcb,'tcpopup'))
      |     case 'IEC Standard Inverse'
      |         title('IEC Standard Inverse');
      |         set(gca, 'YTick', (1:10));
      |         ylim([0.1 10]);
      |     case 'IEC Very Inverse'
      |         title('IEC Very Inverse');
      |         set(gca, 'YTick', (1:2:15));
      |         ylim([0.01 15]);
      |     case 'IEC Long Time Inverse'
      |         title('IEC Long Time Inverse');
      |         set(gca, 'YTick', (0:20:120));
      |         ylim([0.1 120]);
      |     case 'IEC Extremely Inverse'
      |         title('IEC Extremely Inverse');
      |         set(gca, 'YTick', (0:5:30));
      |         ylim([0.01 30]);
      |     case 'IEC Ultra Inverse'
      |         title('IEC Ultra Inverse');
      |         set(gca, 'YTick', (0:20:100));
      |         ylim([0.01 100]);
      |     case 'IEEE Moderately Inverse'
      |         title('IEEE Moderately Inverse');
      |         set(gca, 'YTick', (1:5));
      |         ylim([0.01 5]);
      |     case 'IEEE Very Inverse'
      |         title('IEEE Very Inverse');
      |         set(gca, 'YTick', (1:10));
      |         ylim([0.01 10]);
      |     case 'IEEE Extremely Inverse'
      |         title('IEEE Extremely Inverse');
      |         set(gca, 'YTick', (1:10));
      |         ylim([0.01 10]);
      | end
      | 
      | set(gca, 'XTick', [1:10 20]);
      | xlim([1 30]);
      | xlabel('Current (Multiples of Plug Setting)');
      | ylabel('Operating Time (sec)');
      | grid on;
      mask DialogControl RMS Prompt: RMS Current Measurement
      mask Display:
      | disp('(51)');
      | port_label('input', 1, 'I');
      | port_label('output', 1, 'trip');
      | port_label('output', 2, 'OT');
  Display : Display
  Three-Phase V-I Measurement : powerlib/Measurements/Three-Phase V-I Measurement  VoltageMeasurement=no  SetLabelV=off  LabelV=Vabc  Vpu=off  VpuLL=off  CurrentMeasurement=yes  SetLabelI=off  LabelI=Iabc  Ipu=off  Pbase=100e6  Vbase=500e3  OutputType=Complex  PhasorSimulation=off  PSBequivalent=0
      settings: SourceProductName=Simscape Electrical
  Three-Phase Breaker : powerlib/Elements/Three-Phase Breaker  InitialState=closed  SwitchA=on  SwitchB=on  SwitchC=on  SwitchTimes="[1/60  5/60]"  External=on  BreakerResistance=0.001  SnubberResistance=1e6  SnubberCapacitance=inf  Measurements=None
      settings: SourceProductName=Simscape Electrical
  A : PMIOPort  Side=Left
  a : PMIOPort  Port=2  Side=Right
  B : PMIOPort  Port=3  Side=Left
  b : PMIOPort  Port=4  Side=Right
  C : PMIOPort  Port=5  Side=Left
  c : PMIOPort  Port=6  Side=Right
  tag scope: PV_B=global
  wires:
  Three-Phase V-I Measurement/1 -> AC Time Overcurrent Relay2/1(I)  "Iabc"
  AC Time Overcurrent Relay2/2(OT) -> Display/1
  AC Time Overcurrent Relay2/1(C.B) -> [PV_B], Three-Phase Breaker/1  "Relay C"
  connections:
  Three-Phase Breaker/RConn2 -- Three-Phase V-I Measurement/LConn2
  Three-Phase V-I Measurement/RConn2 -- b/RConn1
  Three-Phase V-I Measurement/LConn1 -- Three-Phase Breaker/RConn1
  Three-Phase Breaker/LConn2 -- B/RConn1
  Three-Phase V-I Measurement/RConn1 -- a/RConn1
  Three-Phase Breaker/RConn3 -- Three-Phase V-I Measurement/LConn3
  Three-Phase Breaker/LConn3 -- C/RConn1
  Three-Phase V-I Measurement/RConn3 -- c/RConn1
  Three-Phase Breaker/LConn1 -- A/RConn1

== system Project_microgrid_2018a/Relay W ==
  AC Time Overcurrent Relay2 : Subsystem  mask(AC Time Overcurrent Relay Block){tcpopup=Definite Minimum Time, k=0, alpha=0.02, B=0, PS=100%, TMS=0.1, TDS=5, CTpri=300, CTsec=5, Freq=60, RMSInit=0}
      mask prompts: tcpopup "Trip Characteristic"; PS "Plug Setting (PS) / Low-set (I >)"; TMS "Time Multiplier Setting (TMS)"; TDS "Time Delay Setting (TDS) in sec"; CTpri "Current Transformer Primary (A)"; CTsec "Current Transformer Secondary (A)"; Freq "Fundamental frequency (Hz):"; RMSInit "Initial RMS value:"
      mask help:
      | AC Time Overcurrent Relay Block developed by Dr Rodney Tan
      | Version 1.0 (Jun 2016)
      |
      | AC Time Overcurrent Relay (ANSI/IEEE C37.2 device number 51) that operates when the current exceeds a predetermined value.
      |
      | This relay operates with either a Definite Minimum Time (DMT) or Inverse Definite Minimum Time (IDMT) characteristic.
      |
      | This relay support both IEC 60255 Standard and IEEE Standard C37.112-1996 IDMT trip characteristic.
      mask Help:
      | <b><u>Block Setting</u></b>
      | <b>Trip Characteristic</b>
      | Relay operation mode selection of Definite Minimum Time (DMT), IEC 60255 Standard or IEEE Standard C37.112-1996 Inverse Definite Minimum Time (IDMT).
      | 
      | <b>Plug-Setting(PS) / Low-set (I >)</b>
      | Specify relay pick-up current based on current transformer rating ranging from 25% to 200% with 25% step interval.
      | 
      | <b>Time Multiplier Setting (TMS)</b>
      | Specify time delay multiplier ranging from 0.05 to 1.0 for IDMT relay operation. This setting will be disabled DMT relay operation mode.
      | 
      | <b>Plot Curve Button</b>
      | Plot current Inverse Definite Minimum Time trip curve.
      | 
      | <b>Time Delay Setting (TDS)</b>
      | Specify time delay ranging from 0.05sec to 99sec for Definite Minimum Time relay operation. This setting will be disabled in IDMT relay operation mode.
      | 
      | <b>Current Transformer Primary (A)</b>
      | Specify current transformer primary in Ampere.
      | 
      | <b>Current Transformer Secondary (A)</b>
      | Specify current transformer secondary in Ampere.
      | 
      | <b>Fundamental Frequency (Hz)</b>
      | Specify the RMS current measurement fundamental frequency, in hertz, of the input signal.
      | 
      | <b>Initial RMS Value</b>
      | Specify the RMS current measurement initial RMS value of the output signal.
      | 
      | <b><u>Block Input Output</u></b>
      | <b>I</b>
      | Current input to the AC time overcurrent relay
      | 
      | <b>trip</b>
      | Trip control signal output (1-0), commonly connected to circuit breaker
      | 
      | <b>OT</b>
      | Relay operating time output
      mask TypeOptions tcpopup: Definite Minimum Time | IEC Standard Inverse | IEC Very Inverse | IEC Long Time Inverse | IEC Extremely Inverse | IEC Ultra Inverse | IEEE Moderately Inverse | IEEE Very Inverse | IEEE Extremely Inverse
      mask Callback tcpopup:
      | switch(get_param(gcb,'tcpopup'))
      |     case 'IEC Standard Inverse'
      |         set_param(gcb,'k','0.14');
      |         set_param(gcb,'alpha','0.02');
      |         set_param(gcb,'B','0');
      |         set_param(gcb,'MaskEnables',{'on','off','off','off',...
      |                   'on','on','off','on','on','on','on'});
      |     case 'IEC Very Inverse'
      |         set_param(gcb,'k','13.5');
      |         set_param(gcb,'alpha','1');
      |         set_param(gcb,'B','0');
      |         set_param(gcb,'MaskEnables',{'on','off','off','off',...
      |                   'on','on','off','on','on','on','on'});
      |     case 'IEC Long Time Inverse'
      |         set_param(gcb,'k','120');
      |         set_param(gcb,'alpha','1');
      |         set_param(gcb,'B','0');
      |         set_param(gcb,'MaskEnables',{'on','off','off','off',...
      |                   'on','on','off','on','on','on','on'});
      |     case 'IEC Extremely Inverse'
      |         set_param(gcb,'k','80');
      |         set_param(gcb,'alpha','2');
      |         set_param(gcb,'B','0');
      |         set_param(gcb,'MaskEnables',{'on','off','off','off',...
      |                   'on','on','off','on','on','on','on'});
      |     case 'IEC Ultra Inverse'
      |         set_param(gcb,'k','315.2');
      |         set_param(gcb,'alpha','2.5');
      |         set_param(gcb,'B','0');
      |         set_param(gcb,'MaskEnables',{'on','off','off','off',...
      |                   'on','on','off','on','on','on','on'});
      |     case 'IEEE Moderately Inverse'
      |         set_param(gcb,'k','0.0515');
      |         set_param(gcb,'alpha','0.02');
      |         set_param(gcb,'B','0.114');
      |         set_param(gcb,'MaskEnables',{'on','off','off','off',...
      |                   'on','on','off','on','on','on','on'});
      |     case 'IEEE Very Inverse'
      |         set_param(gcb,'k','19.61');
      |         set_param(gcb,'alpha','2');
      |         set_param(gcb,'B','0.491');
      |         set_param(gcb,'MaskEnables',{'on','off','off','off',...
      |                   'on','on','off','on','on','on','on'});
      |     case 'IEEE Extremely Inverse'
      |         set_param(gcb,'k','28.2');
      |         set_param(gcb,'alpha','2');
      |         set_param(gcb,'B','0.1217');
      |         set_param(gcb,'MaskEnables',{'on','off','off','off',...
      |                   'on','on','off','on','on','on','on'});
      |     otherwise
      |         set_param(gcb,'k','0');
      |         set_param(gcb,'MaskEnables',{'on','off','off','off',...
      |                   'on','off','on','on','on','on','on'});
      | end
      mask TypeOptions PS: 25% | 50% | 75% | 100% | 125% | 150% | 175% | 200%
      mask TypeOptions TMS: 0.05 | 0.1 | 0.15 | 0.2 | 0.25 | 0.3 | 0.35 | 0.4 | 0.45 | 0.5 | 0.55 | 0.6 | 0.65 | 0.7 | 0.75 | 0.8 | 0.85 | 0.9 | 0.95 | 1.0
      mask Callback TDS:
      | TDS = str2double(get_param(gcb,'TDS'));
      | if (TDS > 99)||(TDS < 0.05)||isnan(TDS)
      |     msgbox('TDS must be in the range of 0.05-99 sec',...
      |     'Invalid Value !','error');
      |     set_param(gcb,'TDS','0.1');
      | end
      mask TypeOptions Freq: Irms/Freq
      mask TypeOptions RMSInit: Irms/RMSInit
      mask DialogControl plotbutton Prompt: Plot Curve
      mask DialogControl plotbutton Callback:
      | % Plotting IDMT Curve
      | TMS = str2num(get_param(gcb,'TMS'));
      | k = str2num(get_param(gcb,'k'));
      | alpha = str2num(get_param(gcb,'alpha'));
      | B = str2num(get_param(gcb,'B'));
      | I = 1:20;
      | td = ((k./((I.^alpha)-1))+B)*TMS;
      | loglog(td);
      | set(gcf, 'Position', [200 150 300 500]);
      | switch(get_param(gcb,'tcpopup'))
      |     case 'IEC Standard Inverse'
      |         title('IEC Standard Inverse');
      |         set(gca, 'YTick', (1:10));
      |         ylim([0.1 10]);
      |     case 'IEC Very Inverse'
      |         title('IEC Very Inverse');
      |         set(gca, 'YTick', (1:2:15));
      |         ylim([0.01 15]);
      |     case 'IEC Long Time Inverse'
      |         title('IEC Long Time Inverse');
      |         set(gca, 'YTick', (0:20:120));
      |         ylim([0.1 120]);
      |     case 'IEC Extremely Inverse'
      |         title('IEC Extremely Inverse');
      |         set(gca, 'YTick', (0:5:30));
      |         ylim([0.01 30]);
      |     case 'IEC Ultra Inverse'
      |         title('IEC Ultra Inverse');
      |         set(gca, 'YTick', (0:20:100));
      |         ylim([0.01 100]);
      |     case 'IEEE Moderately Inverse'
      |         title('IEEE Moderately Inverse');
      |         set(gca, 'YTick', (1:5));
      |         ylim([0.01 5]);
      |     case 'IEEE Very Inverse'
      |         title('IEEE Very Inverse');
      |         set(gca, 'YTick', (1:10));
      |         ylim([0.01 10]);
      |     case 'IEEE Extremely Inverse'
      |         title('IEEE Extremely Inverse');
      |         set(gca, 'YTick', (1:10));
      |         ylim([0.01 10]);
      | end
      | 
      | set(gca, 'XTick', [1:10 20]);
      | xlim([1 30]);
      | xlabel('Current (Multiples of Plug Setting)');
      | ylabel('Operating Time (sec)');
      | grid on;
      mask DialogControl RMS Prompt: RMS Current Measurement
      mask Display:
      | disp('(51)');
      | port_label('input', 1, 'I');
      | port_label('output', 1, 'trip');
      | port_label('output', 2, 'OT');
  Display : Display
  Three-Phase V-I Measurement : powerlib/Measurements/Three-Phase V-I Measurement  VoltageMeasurement=no  SetLabelV=off  LabelV=Vabc  Vpu=off  VpuLL=off  CurrentMeasurement=yes  SetLabelI=off  LabelI=Iabc  Ipu=off  Pbase=100e6  Vbase=500e3  OutputType=Complex  PhasorSimulation=off  PSBequivalent=0
      settings: SourceProductName=Simscape Electrical
  Three-Phase Breaker : powerlib/Elements/Three-Phase Breaker  InitialState=closed  SwitchA=on  SwitchB=on  SwitchC=on  SwitchTimes="[1/60  5/60]"  External=on  BreakerResistance=0.001  SnubberResistance=1e6  SnubberCapacitance=inf  Measurements=None
      settings: SourceProductName=Simscape Electrical
  A : PMIOPort  Side=Left
  a : PMIOPort  Port=2  Side=Right
  B : PMIOPort  Port=3  Side=Left
  b : PMIOPort  Port=4  Side=Right
  C : PMIOPort  Port=5  Side=Left
  c : PMIOPort  Port=6  Side=Right
  tag scope: W_B=global
  wires:
  Three-Phase V-I Measurement/1 -> AC Time Overcurrent Relay2/1(I)  "Iabc"
  AC Time Overcurrent Relay2/2(OT) -> Display/1
  AC Time Overcurrent Relay2/1(C.B) -> [W_B], Three-Phase Breaker/1  "Relay C"
  connections:
  Three-Phase Breaker/RConn2 -- Three-Phase V-I Measurement/LConn2
  Three-Phase V-I Measurement/RConn2 -- b/RConn1
  Three-Phase V-I Measurement/LConn1 -- Three-Phase Breaker/RConn1
  Three-Phase Breaker/LConn2 -- B/RConn1
  Three-Phase V-I Measurement/RConn1 -- a/RConn1
  Three-Phase Breaker/RConn3 -- Three-Phase V-I Measurement/LConn3
  Three-Phase Breaker/LConn3 -- C/RConn1
  Three-Phase V-I Measurement/RConn3 -- c/RConn1
  Three-Phase Breaker/LConn1 -- A/RConn1
